simulink model "simuMotorCapteur"  (R2014a)
settings: Solver=ode45  StartTime=0.0  StopTime=10.0  MaxStep=0.0001  RelTol=1e-3
values from neighbouring files (symbols this model uses):
  contr = param    [parametres.m]
undefined symbols (not defined in the file or in its folder): param
settings Model: Creator=Etienne  LastModifiedBy=Etienne

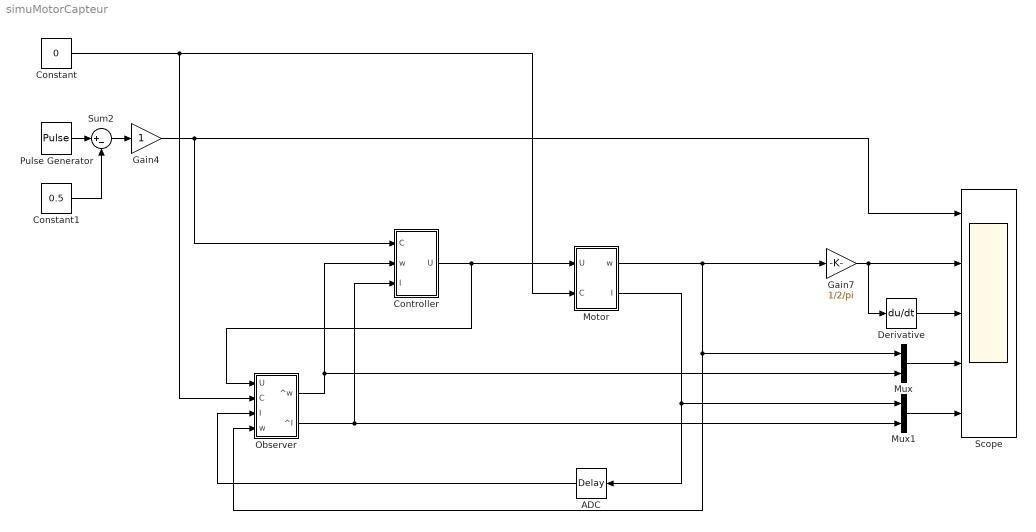
== system simuMotorCapteur ==
  ADC : TransportDelay  DelayTime=78/2/144000
  Constant : Constant  Value=0
  Constant1 : Constant  Value=0.5
  Controller : Subsystem
  Derivative : Derivative
  Gain4 : Gain
  Gain7 : Gain  Gain=1/2/pi
  Motor : Subsystem
  Mux : Mux  Inputs=2
  Mux1 : Mux  Inputs=2
  Observer : Subsystem
  Pulse Generator : DiscretePulseGenerator  PulseType=Time based  Period=1  PulseWidth=50  PhaseDelay=0.25
  Scope : Scope  NumInputPorts=5
      settings: TimeRange=10  YMin=-0.5~-10~-40~-1~-3  YMax=0.5~10~40~1~3  MaxDataPoints=500000
  Sum2 : Sum  Inputs=|+-
  wires:
  Constant/1 -> Motor/2(C), Observer/2(C)
  Motor/1(w) -> Mux/1, Observer/4(w), Gain7/1
  Motor/2(I) -> Mux1/1, ADC/1
  Pulse Generator/1 -> Sum2/1
  Sum2/1 -> Gain4/1
  Constant1/1 -> Sum2/2
  Gain4/1 -> Controller/1(C), Scope/1
  Gain7/1 -> Derivative/1, Scope/2
  Derivative/1 -> Scope/3
  Controller/1(U) -> Observer/1(U), Motor/1(U)
  Observer/2(^I) -> Controller/3(I), Mux1/2
  Observer/1(^w) -> Controller/2(w), Mux/2
  ADC/1 -> Observer/3(I)
  Mux/1 -> Scope/4
  Mux1/1 -> Scope/5

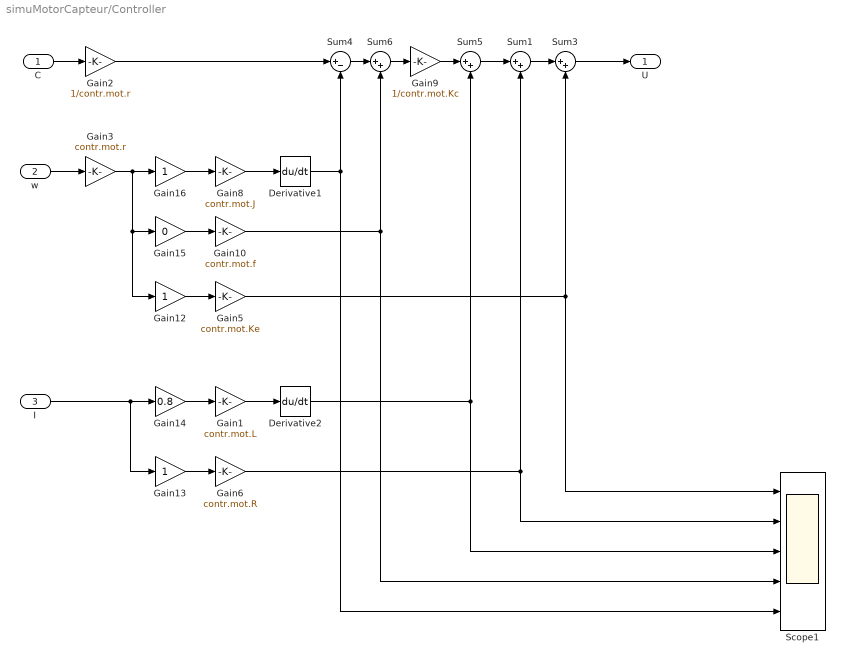
== system simuMotorCapteur/Controller ==
  C : Inport
  w : Inport  Port=2
  I : Inport  Port=3
  Derivative1 : Derivative
  Derivative2 : Derivative
  Gain1 : Gain  Gain=contr.mot.L
  Gain10 : Gain  Gain=contr.mot.f
  Gain12 : Gain
  Gain13 : Gain
  Gain14 : Gain  Gain=0.8
  Gain15 : Gain  Gain=0
  Gain16 : Gain
  Gain2 : Gain  Gain=1/contr.mot.r
  Gain3 : Gain  Gain=contr.mot.r
  Gain5 : Gain  Gain=contr.mot.Ke
  Gain6 : Gain  Gain=contr.mot.R
  Gain8 : Gain  Gain=contr.mot.J
  Gain9 : Gain  Gain=1/contr.mot.Kc
  Scope1 : Scope  NumInputPorts=5
      settings: TimeRange=10  YMin=-30~-5~-1~-1~-0.04  YMax=30~5~1~1~0.04  MaxDataPoints=500000
  Sum{1,3,5..6} (4 alike) : Sum  Inputs=|++
  Sum4 : Sum  Inputs=|+-
  U : Outport
  wires:
  Gain5/1 -> Scope1/1, Sum3/2
  Gain8/1 -> Derivative1/1
  Gain3/1 -> Gain16/1, Gain12/1, Gain15/1
  Gain2/1 -> Sum4/1
  Sum1/1 -> Sum3/1
  Gain6/1 -> Scope1/2, Sum1/2
  Sum3/1 -> U/1
  Sum6/1 -> Gain9/1
  Derivative1/1 -> Scope1/5, Sum4/2
  Derivative2/1 -> Scope1/3, Sum5/2
  Sum5/1 -> Sum1/1
  Gain12/1 -> Gain5/1
  Gain9/1 -> Sum5/1
  Gain1/1 -> Derivative2/1
  Gain15/1 -> Gain10/1
  Gain16/1 -> Gain8/1
  Gain13/1 -> Gain6/1
  Gain14/1 -> Gain1/1
  Sum4/1 -> Sum6/1
  Gain10/1 -> Scope1/4, Sum6/2
  C/1 -> Gain2/1
  w/1 -> Gain3/1
  I/1 -> Gain13/1, Gain14/1

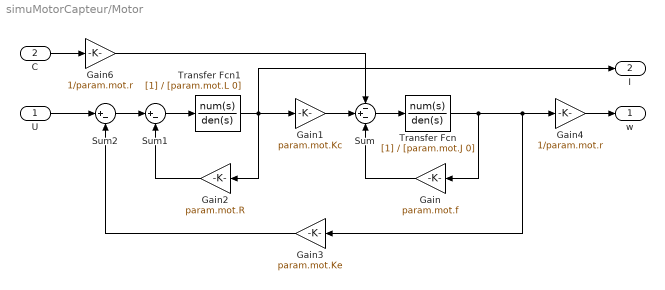
== system simuMotorCapteur/Motor ==
  U : Inport
  C : Inport  Port=2
  Gain : Gain  Gain=param.mot.f
  Gain1 : Gain  Gain=param.mot.Kc
  Gain2 : Gain  Gain=param.mot.R
  Gain3 : Gain  Gain=param.mot.Ke
  Gain4 : Gain  Gain=1/param.mot.r
  Gain6 : Gain  Gain=1/param.mot.r
  Sum : Sum  Inputs=-+-
  Sum1 : Sum  Inputs=|+-
  Sum2 : Sum  Inputs=|+-
  Transfer Fcn : TransferFcn  Denominator=[param.mot.J 0]
  Transfer Fcn1 : TransferFcn  Denominator=[param.mot.L 0]
  w : Outport
  I : Outport  Port=2
  wires:
  Gain1/1 -> Sum/2
  Transfer Fcn/1 -> Gain3/1, Gain4/1, Gain/1
  Gain3/1 -> Sum2/2
  Gain/1 -> Sum/3
  Sum2/1 -> Sum1/1
  Gain2/1 -> Sum1/2
  Sum1/1 -> Transfer Fcn1/1
  U/1 -> Sum2/1
  C/1 -> Gain6/1
  Gain6/1 -> Sum/1
  Gain4/1 -> w/1
  Sum/1 -> Transfer Fcn/1
  Transfer Fcn1/1 -> Gain1/1, I/1, Gain2/1

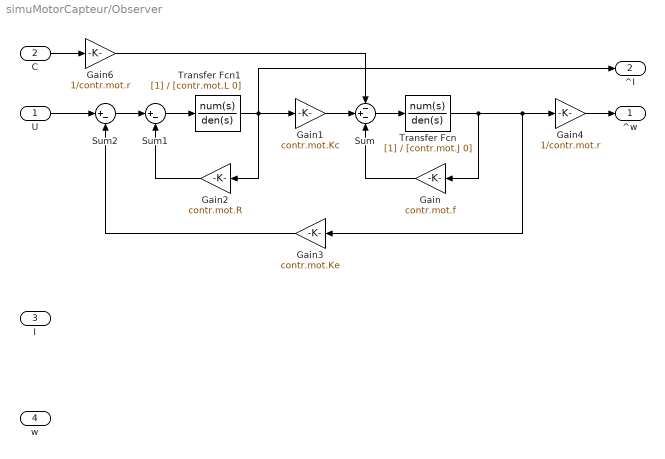
== system simuMotorCapteur/Observer ==
  U : Inport
  C : Inport  Port=2
  I : Inport  Port=3
  w : Inport  Port=4
  Gain : Gain  Gain=contr.mot.f
  Gain1 : Gain  Gain=contr.mot.Kc
  Gain2 : Gain  Gain=contr.mot.R
  Gain3 : Gain  Gain=contr.mot.Ke
  Gain4 : Gain  Gain=1/contr.mot.r
  Gain6 : Gain  Gain=1/contr.mot.r
  Sum : Sum  Inputs=-+-
  Sum1 : Sum  Inputs=|+-
  Sum2 : Sum  Inputs=|+-
  Transfer Fcn : TransferFcn  Denominator=[contr.mot.J 0]
  Transfer Fcn1 : TransferFcn  Denominator=[contr.mot.L 0]
  ^w : Outport
  ^I : Outport  Port=2
  wires:
  Gain1/1 -> Sum/2
  Transfer Fcn/1 -> Gain3/1, Gain4/1, Gain/1
  Gain3/1 -> Sum2/2
  Gain/1 -> Sum/3
  Sum2/1 -> Sum1/1
  Gain2/1 -> Sum1/2
  Sum1/1 -> Transfer Fcn1/1
  U/1 -> Sum2/1
  C/1 -> Gain6/1
  Gain6/1 -> Sum/1
  Gain4/1 -> ^w/1
  Sum/1 -> Transfer Fcn/1
  Transfer Fcn1/1 -> Gain1/1, ^I/1, Gain2/1
